simulink model "RFC_art"  (R2019b)
settings: Solver=FixedStepDiscrete  StartTime=0  StopTime=5  FixedStep=fixedStepSize  MaxStep=0.001  RelTol=1e-3  EnableMultiTasking=on
model workspace (MAT data in the model file):
  Occurrence.FaultRemote = 1
  Occurrence.FaultLow = 2
  Occurrence.FaultLow_2 = 3
  Occurrence.FaultModerate = 4
  Occurrence.FaultModerate_2 = 5
  Occurrence.FaultModerate_3 = 6
  Occurrence.FaultHigh = 7
  Occurrence.FaultHigh_2 = 8
  Occurrence.Tolerance = 9
  Occurrence.OK = 10
  Partitions.Last = ''
  Partitions.All = '*'
  Severity.OK = 0
  Severity.Warn = 1
  Severity.VeryMinor = 2
  Severity.Minor = 3
  Severity.VeryLow = 4
  Severity.Low = 5
  Severity.Moderate = 6
  Severity.High = 7
  Severity.VeryHigh = 8
  Severity.HazardousWithWarning = 9
  Severity.HazardousNoWarning = 10
  Severity.Error = 11
  Severity.ErrorFatal = 20
  block : handle (value not decoded)
  t = 0
  time = 0
undefined symbols (not defined in the file): artificial_AFE_RFC_constant, artificial_RFC_time
settings Model: RequirementInfo={} %GIDa_2eec5742_b109_443f_bad2_42d52c6309f7  conn_id=-1  report_delay=1  Creator=aande176  LastModifiedBy=JEDDELAN
settings SolverCC: AutoInsertRateTranBlk=on
settings DataIOCC: ExternalInput=[],CPSRSts__CPSRSts,[],[],[],[],[],[],[],LvTestSts__LvTestSts,IsgPwrLimMin__IsgPwrLimMin,[],IsgPwrLimMax__IsgPwrLimMax,TqAvlIntFromIfCpt__TqAvlIntFromIfCpt,[],[],[],[],[],TqAllwdInt__TqAllwdInt,[],[],[],[],[],[],[],HvBattUDynMaxLim__HvBattUDynMaxLim,[],HvBattUDynMinLim__HvBattUDynMinLim,[],InitCmpl__InitCmpl,[],[],[],[],[],[],[],[],[],[],[],HvTestSts__HvTestSts,[],[],[],IsgModReq__IsgModReq,[],[],[],[],[],[],[],[],[],[],[],[],[],[],[],[],[],EngSt1WdSts__EngSt1WdSts__IsUpdated,IsgSpdReq__IsgSpdReq__IsUpdated,IsgModReq__IsgModReq__IsUpdated,HvSysRlySts__HvSysRlySts__IsUpdated,HvSysRlySts_toController,[],[],[],[],ImobPrpsnAllwd__ImobPrpsnAllwd__dummy,[],[],[],[],ImobTurnOffAllwd__ImobTurnOffAllwd__dummy,[],[],[],No_GearEven,B_CloseClutchOdd,B_CloseClutchEven,[],[],[],B_EnableVSpAct,V_Vehicle_SetPoint_mps,[]  SaveFormat=StructureWithTime  SaveOutput=off  SaveTime=off  ReturnWorkspaceOutputs=off  SignalLoggingName=slunit_logdata
settings OptimizationCC: DefaultParameterBehavior=Inlined  ExpressionDepthLimit=2147483647  LifeSpan=Inf
settings DebuggingCC: RTPrefix=warning  AlgebraicLoopMsg=error  CheckSSInitialOutputMsg=off  SolverPrmCheckMsg=warning  IntegerOverflowMsg=none  ParameterPrecisionLossMsg=none  FcnCallInpInsideContextMsg=warning  BusObjectLabelMismatch=error  ModelReferenceDataLoggingMessage=none  StateNameClashWarn=warning  SFUnexpectedBacktrackingDiag=warning  SFNoUnconditionalDefaultTransitionDiag=warning  SFExecutionAtInitializationDiag=none  IntegerSaturationMsg=none  ArithmeticOperatorsInVariantConditions=warning
settings HardwareCC: ProdBitPerLong=64  ProdHWDeviceType=Intel->x86-64
settings ModelReferenceCC: UpdateModelReferenceTargets=AssumeUpToDate  PropagateSignalLabelsOutOfModel=off
settings SFSimCC: SimUseLocalCustomCode=off  SimGenImportedTypeDefs=on  CustomCodeUndefinedFunction=UseInterfaceOnly
settings RTWCC: RTWUseLocalCustomCode=off  RTWUseSimCustomCode=on
settings CodeAppCC: StateflowObjectComments=on
settings GRTTargetCC: TargetLangStandard=C89/C90 (ANSI)  GeneratePreprocessorConditionals=Disable all  CombineOutputUpdateFcns=off  MatFileLogging=off  GRTInterface=on
settings ConfigComp: CovScope=Subsystem  CovPath=RequirementsEvaluation/AvailableTorque  CovMetricSettings=dcw  CovHTMLOptions=-sRT=1 -aTS=1 -bRG=1 -bTC=1 -hTR=0 -nFC=0 -scm=1 -bcm=1 -xEv=0  CovHtmlReporting=on  CovSaveCumulativeToWorkspaceVar=on  CovSaveSingleToWorkspaceVar=on  CovExternalEMLEnable=off

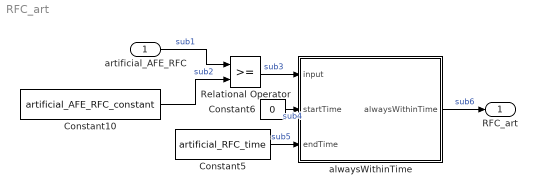
== system RFC_art ==
  artificial_AFE_RFC : Inport
  Constant10 : Constant  Value=artificial_AFE_RFC_constant
  Constant5 : Constant  Value=artificial_RFC_time
  Constant6 : Constant  Value=0
  Relational Operator : RelationalOperator  OutDataTypeStr=boolean  RndMeth=Simplest
  alwaysWithinTime : Subsystem
      settings: CopyFcn=set_param(gcbh,'LinkStatus','none');
  RFC_art : Outport  OutDataTypeStr=boolean  PortDimensions=1  VectorParamsAs1DForOutWhenUnconnected=off
  wires:
  artificial_AFE_RFC/1 -> Relational Operator/1  "sub1"
  Constant10/1 -> Relational Operator/2  "sub2"
  alwaysWithinTime/1(alwaysWithinTime) -> RFC_art/1  "sub6"
  Constant5/1 -> alwaysWithinTime/3(endTime)  "sub5"
  Constant6/1 -> alwaysWithinTime/2(startTime)  "sub4"
  Relational Operator/1 -> alwaysWithinTime/1(input)  "sub3"

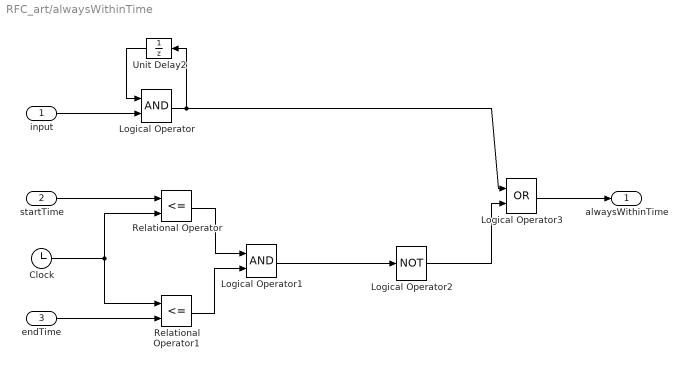
== system RFC_art/alwaysWithinTime ==
  input : Inport
  startTime : Inport  Port=2
  endTime : Inport  Port=3
  Clock : Clock
  Logical Operator : Logic  AllPortsSameDT=off  OutDataTypeStr=boolean
  Logical Operator1 : Logic  AllPortsSameDT=off  OutDataTypeStr=boolean
  Logical Operator2 : Logic  Operator=NOT  AllPortsSameDT=off  OutDataTypeStr=boolean
  Logical Operator3 : Logic  Operator=OR  AllPortsSameDT=off  OutDataTypeStr=boolean
  Relational Operator : RelationalOperator  Operator=<=  OutDataTypeStr=boolean  RndMeth=Simplest
  Relational Operator1 : RelationalOperator  Operator=<=  OutDataTypeStr=boolean  RndMeth=Simplest
  Unit Delay2 : UnitDelay  InitialCondition=1  SampleTime=-1  HasFrameUpgradeWarning=on
  alwaysWithinTime : Outport  VectorParamsAs1DForOutWhenUnconnected=off
  wires:
  startTime/1 -> Relational Operator/1
  Unit Delay2/1 -> Logical Operator/1
  input/1 -> Logical Operator/2
  Logical Operator/1 -> Logical Operator3/1, Unit Delay2/1
  Clock/1 -> Relational Operator1/1, Relational Operator/2
  endTime/1 -> Relational Operator1/2
  Relational Operator1/1 -> Logical Operator1/2
  Relational Operator/1 -> Logical Operator1/1
  Logical Operator1/1 -> Logical Operator2/1
  Logical Operator2/1 -> Logical Operator3/2
  Logical Operator3/1 -> alwaysWithinTime/1
